simulink model "model_nonlinear_bike_closed_loop"  (R2018b)
settings: Solver=VariableStepAuto  StartTime=0.0  StopTime=60  RelTol=1e-3
values from neighbouring files (symbols this model uses):
  bike =     [bike.mat]    (also in modelconfig.mat)
  controller =     [modelconfig.mat]
  model_settings =     [modelconfig.mat]
  parameters =     [modelconfig.mat]
  state_space =     [modelconfig.mat]
undefined symbols (not defined in the file or in its folder): Continuous, Noise, observer, Time
libraries: dspindex x1, sharedTrackingLibrary x1, ctrlSharedLib x1
settings Model: Creator=micha  LastModifiedBy=mekat

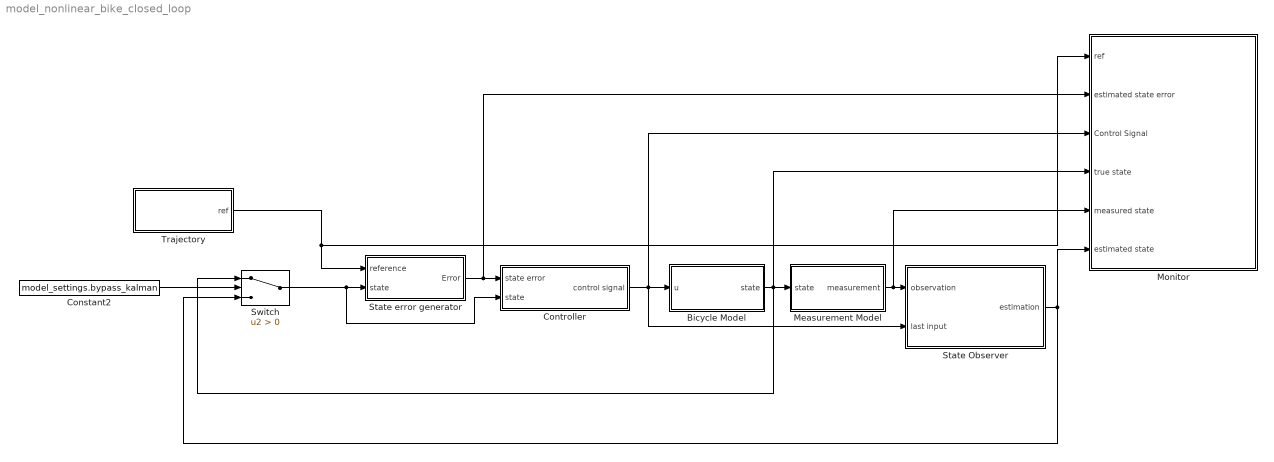
== system model_nonlinear_bike_closed_loop ==
  Bicycle Model : Subsystem
  Constant2 : Constant  Value=model_settings.bypass_kalman
  Controller : Subsystem
  Measurement Model : Subsystem
  Monitor : Subsystem
  State Observer : Subsystem
  State error generator : Subsystem
  Switch : Switch  Criteria=u2 > Threshold
  Trajectory : Subsystem
  wires:
  Bicycle Model/1(state) -> Switch/1, Monitor/4(true state), Measurement Model/1(state)
  Measurement Model/1(measurement) -> Monitor/5(measured state), State Observer/1(observation)
  Controller/1(control signal) -> Bicycle Model/1(u), State Observer/2(last input), Monitor/3(Control Signal)
  State Observer/1(estimation) -> Monitor/6(estimated state), Switch/3
  State error generator/1(Error) -> Controller/1(state error), Monitor/2(estimated state error)
  Trajectory/1(ref) -> State error generator/1(reference), Monitor/1(ref)
  Constant2/1 -> Switch/2
  Switch/1 -> Controller/2(state), State error generator/2(state)

== system model_nonlinear_bike_closed_loop/Bicycle Model ==
  u : Inport
  Constant : Constant  Commented=on  Value=model_settings.limit_model_states
  Nonlinear Model : Subsystem  Commented=on
  Nonlinear Model with Limits : Subsystem
  Switch : Switch  Commented=on  Criteria=u2 > Threshold
  state : Outport
  wires:
  Nonlinear Model with Limits/1(state) -> state/1
  Constant/1 -> Switch/2
  Switch/1 -> ?
  u/1 -> Nonlinear Model with Limits/1(u)

== system model_nonlinear_bike_closed_loop/Controller ==
  state error : Inport
  state : Inport  Port=2
  Constant : Constant  Value=model_settings.use_static_controller
  Dynamic controller : Subsystem
  Static controller : Subsystem
  Switch : Switch  Criteria=u2 > Threshold
  control signal : Outport
  wires:
  state error/1 -> Static controller/1(In1), Dynamic controller/1(stateError)
  Static controller/1(Out1) -> Switch/1
  Dynamic controller/1(control signal) -> Switch/3
  Switch/1 -> control signal/1
  Constant/1 -> Switch/2
  state/1 -> Dynamic controller/2(state)

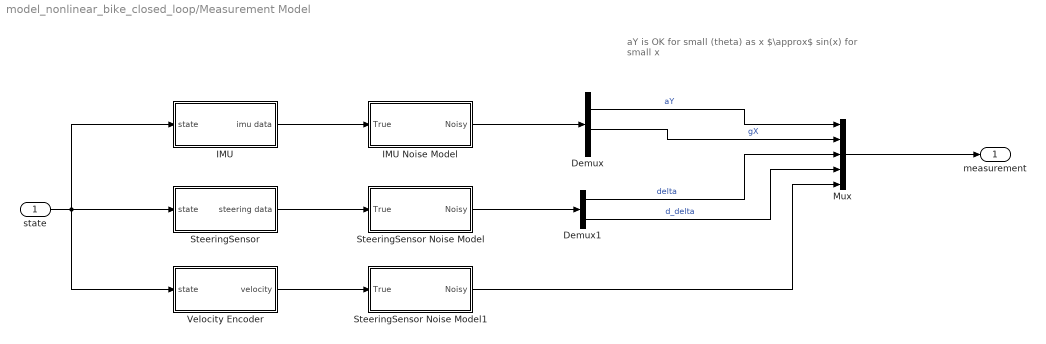
== system model_nonlinear_bike_closed_loop/Measurement Model ==
  note: aY is OK for small (theta) as x $\approx$ sin(x) for small x
  state : Inport
  Demux : Demux  Outputs=6
  Demux1 : Demux  Outputs=2
  IMU : Subsystem
  IMU Noise Model : Subsystem
  Mux : Mux  Inputs=5
  SteeringSensor : Subsystem
  SteeringSensor Noise Model : Subsystem
  SteeringSensor Noise Model1 : Subsystem
  Velocity Encoder : Subsystem
  measurement : Outport
  wires:
  state/1 -> IMU/1(state), Velocity Encoder/1(state), SteeringSensor/1(state)
  IMU/1(imu data) -> IMU Noise Model/1(True)
  SteeringSensor/1(steering data) -> SteeringSensor Noise Model/1(True)
  Demux/4 -> Mux/2  "gX"
  Demux/2 -> Mux/1  "aY"
  Demux1/1 -> Mux/3  "delta"
  Demux1/2 -> Mux/4  "d_delta"
  Mux/1 -> measurement/1
  IMU Noise Model/1(Noisy) -> Demux/1
  SteeringSensor Noise Model/1(Noisy) -> Demux1/1
  Velocity Encoder/1(velocity) -> SteeringSensor Noise Model1/1(True)
  SteeringSensor Noise Model1/1(Noisy) -> Mux/5

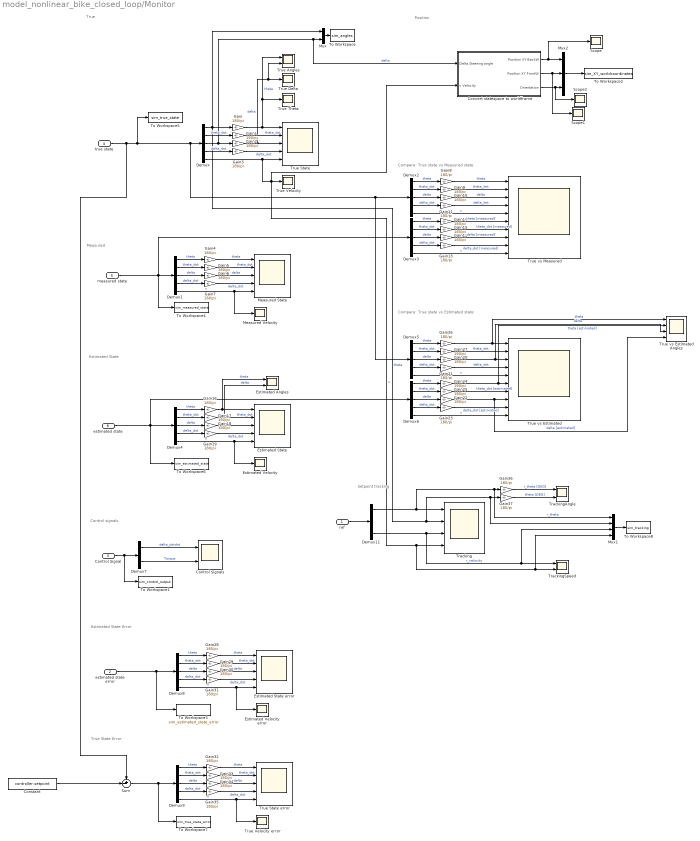
== system model_nonlinear_bike_closed_loop/Monitor ==
  note: Setpoint tracking
  note: Position
  note: Control signals
  note: Estimated State
  note: Compare: True state vs Measured state
  note: True
  note: Measured
  note: Compare: True state vs Estimated state
  note: Estimated State Error
  note: True State Error
  ref : Inport
  estimated state error : Inport  Port=2
  Control Signal : Inport  Port=3
  true state : Inport  Port=4
  measured state : Inport  Port=5
  estimated state : Inport  Port=6
  Constant : Constant  Value=controller.setpoint
  Control Signals : Scope  NumInputPorts=2
  Convert statespace to worldframe : Subsystem
  Demux{,1..6,8..9,11} (10 alike) : Demux  Outputs=5
  Demux7 : Demux  Outputs=2
  Estimated Angles : Scope  NumInputPorts=2
  Estimated State : Scope  NumInputPorts=5
  Estimated State error : Scope  NumInputPorts=5
  Estimated Velocity : Scope
  Estimated Velocity error : Scope
  Gain{,1..37} (38 alike) : Gain  Gain=180/pi
  Measured State : Scope  NumInputPorts=5
  Measured Velocity : Scope
  Mux : Mux  Inputs=2
  Mux1 : Mux
  Mux2 : Mux  Inputs=3
  Scope : Scope
  Scope1 : Scope
  Scope2 : Scope
  Sum : Sum  Inputs=+-|
  To Workspace : ToWorkspace  VariableName=sim_angles  SaveFormat=Structure With Time  SampleTime=-1
  To Workspace1 : ToWorkspace  VariableName=sim_control_output  SaveFormat=Structure With Time  SampleTime=-1
  To Workspace2 : ToWorkspace  VariableName=sim_XY_worldcoordinates  SaveFormat=Structure With Time  SampleTime=-1
  To Workspace3 : ToWorkspace  VariableName=sim_estimated_state_error  SaveFormat=Structure With Time  SampleTime=-1
  To Workspace4 : ToWorkspace  VariableName=sim_measured_state  SaveFormat=Structure With Time  SampleTime=-1
  To Workspace5 : ToWorkspace  VariableName=sim_true_state  SaveFormat=Structure With Time  SampleTime=-1
  To Workspace6 : ToWorkspace  VariableName=sim_estimated_state  SaveFormat=Structure With Time  SampleTime=-1
  To Workspace7 : ToWorkspace  VariableName=sim_true_state_error  SaveFormat=Structure With Time  SampleTime=-1
  To Workspace8 : ToWorkspace  VariableName=sim_tracking  SaveFormat=Structure With Time  SampleTime=-1
  Tracking : Scope  NumInputPorts=4
  TrackingAngle : Scope  NumInputPorts=2
  TrackingSpeed : Scope  NumInputPorts=2
  True Angles : Scope  NumInputPorts=2
  True Delta : Scope
  True State : Scope  NumInputPorts=5
  True State error : Scope  NumInputPorts=5
  True Theta : Scope
  True Velocity : Scope
  True Velocity error : Scope
  True vs Estimated : Scope  NumInputPorts=10
  True vs Estimated Angles : Scope  NumInputPorts=4
  True vs Measured : Scope  NumInputPorts=10
  wires:
  Demux/3 -> Convert statespace to worldframe/1(Delta Steering angle), Mux/2, Gain2/1  "delta"
  Gain3/1 -> True State/4  "delta_dot"
  Demux/4 -> Gain3/1  "delta_dot"
  Demux/2 -> Gain1/1  "theta_dot"
  Demux/5 -> Mux1/4, TrackingSpeed/2, Tracking/4, Convert statespace to worldframe/2(v Velocity), True Velocity/1, True State/5  "v"
  Gain/1 -> True Angles/1, True Theta/1, True State/1  "theta"
  Gain1/1 -> True State/2  "theta_dot"
  Demux/1 -> Mux1/2, Gain37/1, Tracking/2, Mux/1, Gain/1  "theta"
  Gain2/1 -> True Angles/2, True Delta/1, True State/3  "delta"
  Demux1/4 -> Gain7/1  "delta_dot"
  Demux1/3 -> Gain6/1  "delta"
  Gain7/1 -> Measured State/4  "delta_dot"
  Gain6/1 -> Measured State/3  "delta"
  Gain4/1 -> Measured State/1  "theta"
  Demux1/5 -> Measured Velocity/1, Measured State/5  "v"
  Demux1/1 -> Gain4/1  "theta"
  Demux1/2 -> Gain5/1  "theta_dot"
  Gain5/1 -> Measured State/2  "theta_dot"
  Demux2/4 -> Gain11/1  "delta_dot"
  Demux2/3 -> Gain10/1  "delta"
  Gain11/1 -> True vs Measured/4  "delta_dot"
  true state/1 -> Sum/1, To Workspace5/1, Demux5/1, Demux2/1, Demux/1
  Gain10/1 -> True vs Measured/3  "delta"
  Gain8/1 -> True vs Measured/1  "theta"
  Demux2/5 -> True vs Measured/5  "v"
  Demux2/1 -> Gain8/1  "theta"
  Demux2/2 -> Gain9/1  "theta_dot"
  Gain9/1 -> True vs Measured/2  "theta_dot"
  measured state/1 -> To Workspace4/1, Demux3/1, Demux1/1
  Gain14/1 -> True vs Measured/6  "theta [measured]"
  Gain13/1 -> True vs Measured/9  "delta_dot [measured]"
  Demux3/3 -> Gain12/1  "delta"
  Gain12/1 -> True vs Measured/8  "delta [measured]"
  Gain15/1 -> True vs Measured/7  "theta_dot [measured]"
  Demux3/4 -> Gain13/1  "delta_dot"
  Demux3/2 -> Gain15/1  "theta_dot"
  Demux3/1 -> Gain14/1  "theta"
  Demux3/5 -> True vs Measured/10  "v"
  Gain16/1 -> Estimated Angles/1, Estimated State/1  "theta"
  Gain19/1 -> Estimated State/4  "delta_dot"
  Demux4/4 -> Gain19/1  "delta_dot"
  Demux4/1 -> Gain16/1  "theta"
  Gain17/1 -> Estimated State/2  "theta_dot"
  Demux4/3 -> Gain18/1  "delta"
  Demux4/5 -> Estimated Velocity/1, Estimated State/5  "v"
  Gain18/1 -> Estimated Angles/2, Estimated State/3  "delta"
  Demux4/2 -> Gain17/1  "theta_dot"
  Demux6/1 -> Gain24/1  "theta"
  Demux6/3 -> Gain22/1  "delta"
  Gain24/1 -> True vs Estimated Angles/2, True vs Estimated/6  "theta [estimated]"
  Gain20/1 -> True vs Estimated Angles/3, True vs Estimated/3  "delta"
  Gain21/1 -> True vs Estimated/4  "delta_dot"
  Gain26/1 -> True vs Estimated/1, True vs Estimated Angles/1  "theta"
  Demux5/5 -> True vs Estimated/5  "v"
  Gain27/1 -> True vs Estimated/2  "theta_dot"
  Demux5/3 -> Gain20/1  "delta"
  Demux5/4 -> Gain21/1  "delta_dot"
  Demux5/2 -> Gain27/1  "theta_dot"
  Demux6/5 -> True vs Estimated/10  "v"
  Demux5/1 -> Gain26/1  "theta"
  Gain22/1 -> True vs Estimated Angles/4, True vs Estimated/8  "delta [estimated]"
  Demux6/4 -> Gain23/1  "delta_dot"
  Gain25/1 -> True vs Estimated/7  "theta_dot [estimated]"
  Demux6/2 -> Gain25/1  "theta_dot"
  Gain23/1 -> True vs Estimated/9  "delta_dot [estimated]"
  estimated state/1 -> Demux6/1, To Workspace6/1, Demux4/1
  Control Signal/1 -> To Workspace1/1, Demux7/1
  Demux7/1 -> Control Signals/1  "delta_dotdot"
  Demux7/2 -> Control Signals/2  "Torque"
  Gain30/1 -> Estimated State error/3  "delta"
  Demux8/2 -> Gain29/1  "theta_dot"
  Demux8/3 -> Gain30/1  "delta"
  Gain31/1 -> Estimated State error/4  "delta_dot"
  Demux8/5 -> Estimated Velocity error/1, Estimated State error/5  "v"
  Demux8/1 -> Gain28/1  "theta"
  Demux8/4 -> Gain31/1  "delta_dot"
  Gain28/1 -> Estimated State error/1  "theta"
  estimated state error/1 -> To Workspace3/1, Demux8/1
  Gain29/1 -> Estimated State error/2  "theta_dot"
  Demux9/1 -> Gain32/1  "theta"
  Demux9/4 -> Gain35/1  "delta_dot"
  Gain32/1 -> True State error/1  "theta"
  Demux9/5 -> True Velocity error/1, True State error/5  "v"
  Sum/1 -> To Workspace7/1, Demux9/1
  Demux9/2 -> Gain33/1  "theta_dot"
  Gain33/1 -> True State error/2  "theta_dot"
  Gain35/1 -> True State error/4  "delta_dot"
  Demux9/3 -> Gain34/1  "delta"
  Gain34/1 -> True State error/3  "delta"
  Constant/1 -> Sum/2
  Mux/1 -> To Workspace/1
  ref/1 -> Demux11/1
  Demux11/1 -> Mux1/1, Gain36/1, Tracking/1  "r_theta"
  Demux11/5 -> Mux1/3, TrackingSpeed/1, Tracking/3  "r_velocity"
  Gain36/1 -> TrackingAngle/1  "r_theta [DEG]"
  Gain37/1 -> TrackingAngle/2  "theta [DEG]"
  Mux1/1 -> To Workspace8/1
  Convert statespace to worldframe/3(Orientation) -> Scope2/1, Mux2/3
  Convert statespace to worldframe/2(Position XY FrontW) -> Scope1/1, Mux2/2
  Convert statespace to worldframe/1(Position XY BackW) -> Scope/1, Mux2/1
  Mux2/1 -> To Workspace2/1

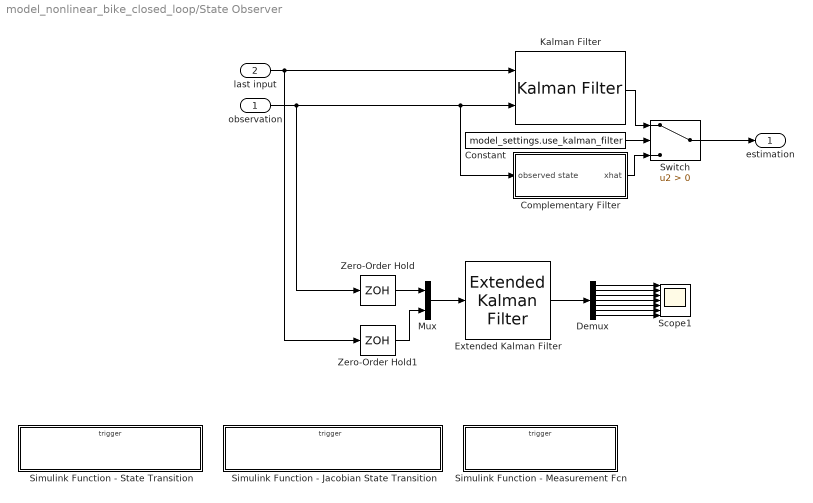
== system model_nonlinear_bike_closed_loop/State Observer ==
  observation : Inport
  last input : Inport  Port=2
  Complementary Filter : Subsystem
  Constant : Constant  Value=model_settings.use_kalman_filter
  Demux : Demux  Outputs=7
  Extended Kalman Filter : sharedTrackingLibrary/Extended Kalman Filter  StateTransitionFcn=stateTransitionFcn  HasStateTransitionJacobianFcn=on  StateTransitionJacobianFcn=JacobianStateTransitionFcn  HasAdditiveProcessNoise=Additive  ProcessNoise=EKF.Noise.stateEstimate  HasTimeVaryingProcessNoise=off  HasStateTransitionFcnExtraArgument=0  InitialState=EKF.InitialPoint  InitialStateCovariance=EKF.Noise.InitialPoint  MeasurementFcn1=measurementFcn  HasMeasurementJacobianFcn1=off  HasMeasurementEnablePort1=off  HasAdditiveMeasurementNoise1=Additive  MeasurementNoise1=EKF.Noise.measurement  HasTimeVaryingMeasurementNoise1=off  HasMeasurementFcnExtraArgument1=0  MeasurementFcn2=myMeasurementFcn  HasMeasurementJacobianFcn2=off  HasMeasurementEnablePort2=off  HasAdditiveMeasurementNoise2=Additive  MeasurementNoise2=1  HasTimeVaryingMeasurementNoise2=off  HasMeasurementFcnExtraArgument2=0  MeasurementFcn3=myMeasurementFcn  HasMeasurementJacobianFcn3=off  HasMeasurementEnablePort3=off  HasAdditiveMeasurementNoise3=Additive  MeasurementNoise3=1  HasTimeVaryingMeasurementNoise3=off  HasMeasurementFcnExtraArgument3=0  MeasurementFcn4=myMeasurementFcn  HasMeasurementJacobianFcn4=off  HasMeasurementEnablePort4=off  HasAdditiveMeasurementNoise4=Additive  MeasurementNoise4=1  HasTimeVaryingMeasurementNoise4=off  HasMeasurementFcnExtraArgument4=0  MeasurementFcn5=myMeasurementFcn  HasMeasurementJacobianFcn5=off  HasMeasurementEnablePort5=off  HasAdditiveMeasurementNoise5=Additive  MeasurementNoise5=1  HasTimeVaryingMeasurementNoise5=off  HasMeasurementFcnExtraArgument5=0  EnableMultirate=off  StateTransitionFcnSampleTime=1  MeasurementFcn1SampleTime=1  MeasurementFcn2SampleTime=1  MeasurementFcn3SampleTime=1  MeasurementFcn4SampleTime=1  MeasurementFcn5SampleTime=1  UseCurrentEstimator=on  OutputStateCovariance=off  DataType=double  SampleTime=parameters.Ts  NumberOfMeasurements=1
      settings: SourceProductName=Control System Toolbox  SourceProductBaseCode=CT
  Kalman Filter : ctrlSharedLib/Kalman Filter  TimeDomain=Continuous-Time  UseCurrentEstimator=on  ModelSource=Individual A, B, C, D matrices  ModelSourceVariable=ss(0.95,1,1,0,1)  A=state_space.A  B=state_space.B  C=state_space.C  D=state_space.D  NumberOfStates=1  NumberOfInputs=1  NumberOfOutputs=1  InitialEstimateSource=Dialog  X0=state_space.x0  P0=10  UseK=off  UseGH=off  NumberOfProcessNoiseInputs=1  G=1  TimeInvariantG=on  H=0  TimeInvariantH=on  Q=observer.Q  TimeInvariantQ=on  R=observer.R  TimeInvariantR=on  N=0  TimeInvariantN=on  AddInputPort=on  AddEnablePort=off  OutputEstimatedY=off  OutputP=off  Ts=-1
      settings: SourceProductBaseCode=CT
  Mux : Mux  Inputs=2
  Scope1 : Scope  NumInputPorts=7
  "Simulink Function - Jacobian State Transition " : Subsystem  TreatAsAtomicUnit=on
  Simulink Function - Measurement Fcn : Subsystem  TreatAsAtomicUnit=on
  Simulink Function - State Transition : Subsystem  TreatAsAtomicUnit=on
  Switch : Switch  Criteria=u2 > Threshold
  Zero-Order Hold : ZeroOrderHold  SampleTime=parameters.Ts
  Zero-Order Hold1 : ZeroOrderHold  SampleTime=parameters.Ts
  estimation : Outport
  wires:
  observation/1 -> Zero-Order Hold/1, Kalman Filter/2, Complementary Filter/1(observed state)
  last input/1 -> Zero-Order Hold1/1, Kalman Filter/1
  Switch/1 -> estimation/1
  Kalman Filter/1 -> Switch/1
  Complementary Filter/1(xhat) -> Switch/3
  Constant/1 -> Switch/2
  Demux/2 -> Scope1/2
  Demux/4 -> Scope1/4
  Demux/5 -> Scope1/5
  Demux/3 -> Scope1/3
  Demux/1 -> Scope1/1
  Extended Kalman Filter/1 -> Demux/1
  Zero-Order Hold/1 -> Mux/1
  Zero-Order Hold1/1 -> Mux/2
  Mux/1 -> Extended Kalman Filter/1
  Demux/6 -> Scope1/6
  Demux/7 -> Scope1/7

== system model_nonlinear_bike_closed_loop/State error generator ==
  reference : Inport
  state : Inport  Port=2
  Sum : Sum  Inputs=|-+
  Error : Outport
  wires:
  reference/1 -> Sum/1
  Sum/1 -> Error/1
  state/1 -> Sum/2

== system model_nonlinear_bike_closed_loop/Trajectory ==
  Clock : Clock
  Constant : Constant  Value=model_settings.SpeedProfile
  Constant1 : Constant  Value=0
  Constant2 : Constant  Value=state_space.x0(5)
  MATLAB Function : MATLAB Function  TreatAsAtomicUnit=on
  Mux : Mux  Inputs=5
  ref : Outport
  wires:
  Mux/1 -> ref/1
  Constant1/1 -> Mux/4, Mux/3, Mux/2, Mux/1
  Clock/1 -> MATLAB Function/1(t)
  MATLAB Function/1(v) -> Mux/5
  Constant/1 -> MATLAB Function/2(t_case)
  Constant2/1 -> MATLAB Function/3(v0)

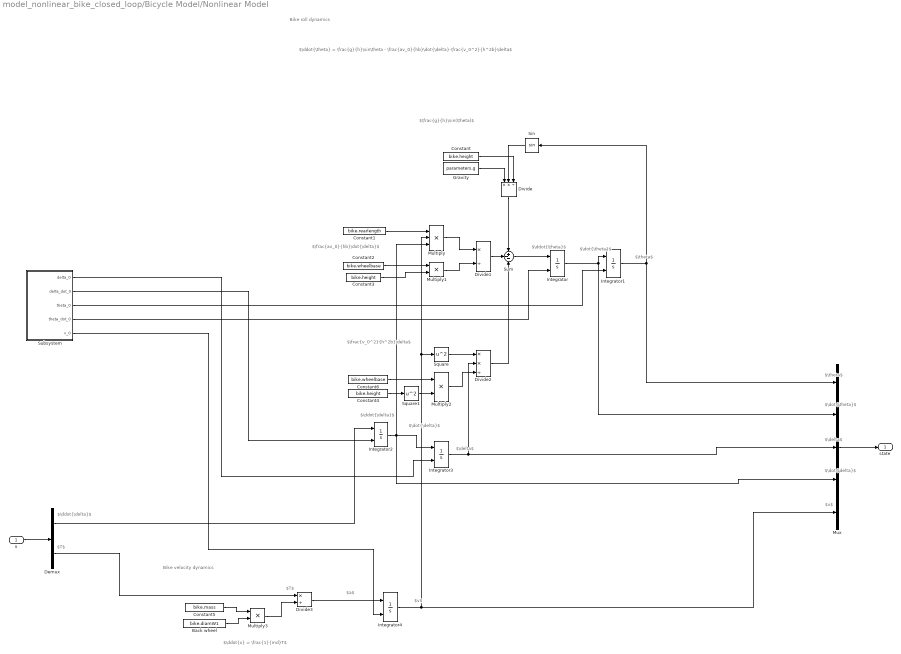
== system model_nonlinear_bike_closed_loop/Bicycle Model/Nonlinear Model ==
  note: Bike velocity dynamics
  note: $\ddot{\theta} = \frac{g}{h}\sin\theta - \frac{av_0}{hb}\dot{\delta}-\frac{v_0^2}{h^2b}\delta$
  note: Bike roll dynamics
  note: $\ddot{x} = \frac{1}{md}T$
  note: $T$
  note: $v$
  note: $a$
  note: $\frac{v_0^2}{h^2b}\delta$
  note: $\frac{g}{h}\sin(\theta)$
  note: $\frac{av_0}{hb}\dot{\delta}$
  note: $\delta$
  note: $\dot{\delta}$
  note: $\ddot{\delta}$
  note: $\theta$
  note: $\dot{\theta}$
  note: $\ddot{\theta}$
  note: $\theta$
  note: $\dot{\theta}$
  note: $\delta$
  note: $\dot{\delta}$
  note: $v$
  note: $\ddot{\delta}$
  note: $T$
  u : Inport
  Back wheel : Constant  Value=bike.diamW1
  Constant : Constant  Value=bike.height
  Constant1 : Constant  Value=bike.rearlength
  Constant2 : Constant  Value=bike.wheelbase
  Constant3 : Constant  Value=bike.height
  Constant4 : Constant  Value=bike.height
  Constant5 : Constant  Value=bike.mass
  Constant6 : Constant  Value=bike.wheelbase
  Demux : Demux  Outputs=2
  Divide : Product  Inputs=**/
  Divide1 : Product  Inputs=*/
  Divide2 : Product  Inputs=**/
  Divide3 : Product  Inputs=*/
  Gravity : Constant  Value=parameters.g
  Integrator{,1..4} (5 alike) : Integrator  InitialConditionSource=external
  Multiply : Product  Inputs=3
  Multiply1 : Product
  Multiply2 : Product
  Multiply3 : Product
  Mux : Mux  Inputs=5
  Sin : Trigonometry
  Square : Math  Operator=square  SaturateOnIntegerOverflow=on
  Square1 : Math  Operator=square  SaturateOnIntegerOverflow=on
  Subsystem : Subsystem
  Sum : Sum  Inputs=+--
  state : Outport
  wires:
  Integrator/1 -> Integrator1/1, Mux/2
  Integrator1/1 -> Mux/1, Sin/1
  Sum/1 -> Integrator/1
  Divide/1 -> Sum/1
  Gravity/1 -> Divide/1
  Sin/1 -> Divide/2
  Constant/1 -> Divide/3
  Demux/1 -> Integrator2/1
  Integrator2/1 -> Integrator3/1, Mux/4, Multiply/3
  Integrator3/1 -> Mux/3, Divide2/2
  Divide1/1 -> Sum/2
  Multiply/1 -> Divide1/1
  Multiply1/1 -> Divide1/2
  Constant1/1 -> Multiply/1
  Constant2/1 -> Multiply1/1
  Constant3/1 -> Multiply1/2
  Divide2/1 -> Sum/3
  Multiply2/1 -> Divide2/3
  Constant4/1 -> Square1/1
  Constant6/1 -> Multiply2/1
  Mux/1 -> state/1
  u/1 -> Demux/1
  Integrator4/1 -> Multiply/2, Square/1, Mux/5
  Square/1 -> Divide2/1
  Square1/1 -> Multiply2/2
  Demux/2 -> Divide3/1
  Multiply3/1 -> Divide3/2
  Constant5/1 -> Multiply3/1
  Back wheel/1 -> Multiply3/2
  Divide3/1 -> Integrator4/1
  Subsystem/3(theta_0) -> Integrator1/2
  Subsystem/4(theta_dot_0) -> Integrator/2
  Subsystem/2(delta_dot_0) -> Integrator2/2
  Subsystem/1(delta_0) -> Integrator3/2
  Subsystem/5(v_0) -> Integrator4/2

== system model_nonlinear_bike_closed_loop/Bicycle Model/Nonlinear Model with Limits ==
  note: $\theta$
  note: $\dot{\theta}$
  note: $\delta$
  note: $\dot{\delta}$
  note: $v$
  note: $\ddot{\delta}$
  note: $T$
  u : Inport
  Demux : Demux  Outputs=2
  Mux : Mux  Inputs=5
  Roll Dynamics : Subsystem
  Velocity Dynamics : Subsystem
  state : Outport
  wires:
  Mux/1 -> state/1
  u/1 -> Demux/1
  Demux/1 -> Roll Dynamics/2(delta_dot_dot)
  Roll Dynamics/1(theta) -> Mux/1
  Roll Dynamics/2(theta_dot) -> Mux/2
  Roll Dynamics/3(delta) -> Mux/3
  Roll Dynamics/4(delta_dot) -> Mux/4
  Velocity Dynamics/1(v) -> Roll Dynamics/1(v), Mux/5
  Demux/2 -> Velocity Dynamics/1(T)

== system model_nonlinear_bike_closed_loop/Controller/Dynamic controller ==
  note: These two blocks implement the same controller.
      | The simulink implementation was made in the hopes that
      | it would be faster.
  stateError : Inport
  state : Inport  Port=2
  Constant : Constant  Value=controller.vmin
  Constant1 : Constant  Value=controller.vmax
  Constant2 : Constant  Value=model_settings.simulink_implementation
  MATLAB Function : MATLAB Function  TreatAsAtomicUnit=on
  Simulink implementation : Subsystem
  Switch : Switch  Criteria=u2 > Threshold
  control signal : Outport
  wires:
  stateError/1 -> Simulink implementation/2(state_error), MATLAB Function/3(state)
  MATLAB Function/1(feedback) -> Switch/3
  Constant/1 -> Simulink implementation/3(vmin), MATLAB Function/1(vmin)
  Constant1/1 -> Simulink implementation/4(vmax), MATLAB Function/2(vmax)
  Constant2/1 -> Switch/2
  Simulink implementation/1(feedback) -> Switch/1
  Switch/1 -> control signal/1
  state/1 -> Simulink implementation/1(state)

== system model_nonlinear_bike_closed_loop/Controller/Static controller ==
  In1 : Inport
  Gain : Gain  Gain=-controller.K  Multiplication=Matrix(K*u)
  Out1 : Outport
  wires:
  Gain/1 -> Out1/1
  In1/1 -> Gain/1

== system model_nonlinear_bike_closed_loop/Measurement Model/IMU ==
  state : Inport
  Accelerometer : Subsystem
  Gyroscope : Subsystem
  Mux : Mux  Inputs=2
  imu data : Outport
  wires:
  state/1 -> Gyroscope/1(state), Accelerometer/1(state)
  Mux/1 -> imu data/1
  Accelerometer/1(acceleration) -> Mux/1  "acc"
  Gyroscope/1(gyro) -> Mux/2  "gyro"

== system model_nonlinear_bike_closed_loop/Measurement Model/IMU Noise Model ==
  note: Generate additive noise
  True : Inport
  Constant1 : Constant  Value=zeros(6,1)
  Constant2 : Constant  Value=model_settings.enable_imu_noise
  Noise Covariance : Gain  Gain=Noise.IMU  Multiplication=Matrix(K*u)
  Random Gaussian : RandomNumber  Seed=round(100000*rand(6,1))  SampleTime=0.02
  Sum : Sum  Inputs=|++
  Switch : Switch  Criteria=u2 > Threshold
  Noisy : Outport
  wires:
  Random Gaussian/1 -> Switch/1
  Switch/1 -> Noise Covariance/1
  Constant2/1 -> Switch/2
  Constant1/1 -> Switch/3
  Noise Covariance/1 -> Sum/2
  True/1 -> Sum/1
  Sum/1 -> Noisy/1

== system model_nonlinear_bike_closed_loop/Measurement Model/SteeringSensor ==
  state : Inport
  Demux : Demux  Outputs=5
  Mux : Mux  Inputs=2
  steering data : Outport
  wires:
  state/1 -> Demux/1
  Mux/1 -> steering data/1
  Demux/3 -> Mux/1  "delta"
  Demux/4 -> Mux/2  "d_delta"

== system model_nonlinear_bike_closed_loop/Measurement Model/SteeringSensor Noise Model ==
  note: Generate additive noise
  True : Inport
  Constant1 : Constant  Value=zeros(2,1)
  Constant2 : Constant  Value=model_settings.enable_encoder_noise
  Noise Covariance : Gain  Gain=Noise.steering_encoder_noise  Multiplication=Matrix(K*u)
  Random Gaussian : RandomNumber  Seed=round(100000*rand(2,1))  SampleTime=0.02
  Sum : Sum  Inputs=-+|
  Switch : Switch  Criteria=u2 > Threshold
  Noisy : Outport
  wires:
  True/1 -> Sum/2
  Switch/1 -> Noise Covariance/1
  Constant1/1 -> Switch/3
  Constant2/1 -> Switch/2
  Random Gaussian/1 -> Switch/1
  Sum/1 -> Noisy/1
  Noise Covariance/1 -> Sum/1

== system model_nonlinear_bike_closed_loop/Measurement Model/SteeringSensor Noise Model1 ==
  note: Generate additive noise
  True : Inport
  Constant1 : Constant  Value=zeros(1,1)
  Constant2 : Constant  Value=model_settings.enable_velocity_noise
  Noise Covariance : Gain  Gain=Noise.velocity_sensor  Multiplication=Matrix(K*u)
  Random Gaussian : RandomNumber  Seed=round(100000*rand(1,1))  SampleTime=0.02
  Sum : Sum  Inputs=-+|
  Switch : Switch  Criteria=u2 > Threshold
  Noisy : Outport
  wires:
  True/1 -> Sum/2
  Switch/1 -> Noise Covariance/1
  Constant1/1 -> Switch/3
  Constant2/1 -> Switch/2
  Random Gaussian/1 -> Switch/1
  Sum/1 -> Noisy/1
  Noise Covariance/1 -> Sum/1

== system model_nonlinear_bike_closed_loop/Measurement Model/Velocity Encoder ==
  state : Inport
  Demux : Demux  Outputs=5
  velocity : Outport
  wires:
  state/1 -> Demux/1
  Demux/5 -> velocity/1

== system model_nonlinear_bike_closed_loop/Monitor/Convert statespace to worldframe ==
  note: This is a forward kinematic system that calculates the
      | velocity in the bikes internal frame and then is
      | transformed (rotated and "translated") into the
      | world frame X and Y.
      | Here to simplify, the orientation is assumed to be
      | the integration of the steering angle.
      | Assumes that bike starts with backwheel in origo and frontwheel on x-axis
  Delta Steering angle : Inport
  v Velocity : Inport  Port=2
  Convert Statespace to World frame : MATLAB Function  TreatAsAtomicUnit=on
  MATLAB Function : MATLAB Function  TreatAsAtomicUnit=on
  Position1 : Integrator  InitialConditionSource=external  InitialCondition=[0,0]'  ContinuousStateAttributes='Position_Global'
  StartingPos Frontwheel : Constant  Value=[bike.wheelbase,0]'
  "orientation " : Integrator  ContinuousStateAttributes='Orientation'
  Position XY BackW : Outport
  Position XY FrontW : Outport  Port=2
  Orientation : Outport  Port=3
  wires:
  "orientation "/1 -> Orientation/1, MATLAB Function/1(orientation), Convert Statespace to World frame/1(orientation_n)
  Delta Steering angle/1 -> Convert Statespace to World frame/2(delta), "orientation "/1
  v Velocity/1 -> Convert Statespace to World frame/3(velocity)
  Convert Statespace to World frame/1(Vel_FW) -> Position1/1
  Position1/1 -> Position XY FrontW/1, MATLAB Function/2(Pos_frontwheel)
  StartingPos Frontwheel/1 -> Position1/2
  MATLAB Function/1(Pos_BW) -> Position XY BackW/1

== system model_nonlinear_bike_closed_loop/State Observer/Complementary Filter ==
  note: $v$
  note: $\dot{\delta}$
  note: $\delta$
  note: $\dot{\theta}$
  note: $\theta$
  observed state : Inport
  Demux : Demux  Outputs=5
  Mux : Mux  Inputs=5
  Subsystem : Subsystem
  Subsystem1 : Subsystem
  xhat : Outport
  wires:
  observed state/1 -> Demux/1
  Demux/2 -> Subsystem/2(obs.rate)
  Demux/3 -> Subsystem1/1(obs.angle)
  Demux/4 -> Subsystem1/2(obs.rate)
  Mux/1 -> xhat/1
  Demux/5 -> Mux/5
  Demux/1 -> Subsystem/1(obs.angle)
  Subsystem/1(est.angle) -> Mux/1
  Subsystem/2(est.rate) -> Mux/2
  Subsystem1/1(est.angle) -> Mux/3
  Subsystem1/2(est.rate) -> Mux/4

== system model_nonlinear_bike_closed_loop/State Observer/Simulink Function - Jacobian State Transition  ==
  JacobianStateTransitionFcn : TriggerPort  TriggerType=function-call  IsSimulinkFunction=on  FunctionName=JacobianStateTransitionFcn  VariantControl=(inherit)
  Demux : Demux  Outputs=7
  MATLAB Function : MATLAB Function  TreatAsAtomicUnit=on
  Mux : Mux  Inputs=3
  Terminator{,1..3} (4 alike) : Terminator
  x : ArgIn  DisableCoverage=on  PortDimensions=7  ArgumentName=x
  A~ : ArgOut  DisableCoverage=on  PortDimensions=[7,7]  ArgumentName=A
  wires:
  x/1 -> Demux/1
  Mux/1 -> MATLAB Function/1(xhat)
  Demux/5 -> Mux/3
  Demux/4 -> Mux/2
  Demux/3 -> Mux/1
  Demux/1 -> Terminator/1
  Demux/2 -> Terminator1/1
  Demux/7 -> Terminator3/1
  Demux/6 -> Terminator2/1
  MATLAB Function/1(A) -> A~/1

== system model_nonlinear_bike_closed_loop/State Observer/Simulink Function - Measurement Fcn ==
  measurementFcn : TriggerPort  TriggerType=function-call  IsSimulinkFunction=on  FunctionName=measurementFcn  VariantControl=(inherit)
  x : ArgIn  DisableCoverage=on  PortDimensions=7  ArgumentName=x
  y : ArgOut  DisableCoverage=on  PortDimensions=7  ArgumentName=y
  wires:
  x/1 -> y/1

== system model_nonlinear_bike_closed_loop/State Observer/Simulink Function - State Transition ==
  stateTransitionFcn : TriggerPort  TriggerType=function-call  IsSimulinkFunction=on  FunctionName=stateTransitionFcn  VariantControl=(inherit)  ShowOutputPort=on  OutputDataType=double
  MATLAB SFunction : MATLAB Function  TreatAsAtomicUnit=on
  x : ArgIn  DisableCoverage=on  PortDimensions=7  ArgumentName=x
  xNext : ArgOut  DisableCoverage=on  PortDimensions=7  ArgumentName=xNext
  wires:
  MATLAB SFunction/1(next_xhat) -> xNext/1
  x/1 -> MATLAB SFunction/1(xhat)

== system model_nonlinear_bike_closed_loop/Bicycle Model/Nonlinear Model/Subsystem ==
  Constant : Constant  Value=state_space.x0(1)
  Constant1 : Constant  Value=state_space.x0(2)
  Constant2 : Constant  Value=state_space.x0(3)
  Constant3 : Constant  Value=state_space.x0(4)
  Constant4 : Constant  Value=state_space.x0(5)
  delta_0 : Outport
  delta_dot_0 : Outport  Port=2
  theta_0 : Outport  Port=3
  theta_dot_0 : Outport  Port=4
  v_0 : Outport  Port=5
  wires:
  Constant/1 -> delta_0/1
  Constant1/1 -> delta_dot_0/1
  Constant2/1 -> theta_0/1
  Constant3/1 -> theta_dot_0/1
  Constant4/1 -> v_0/1

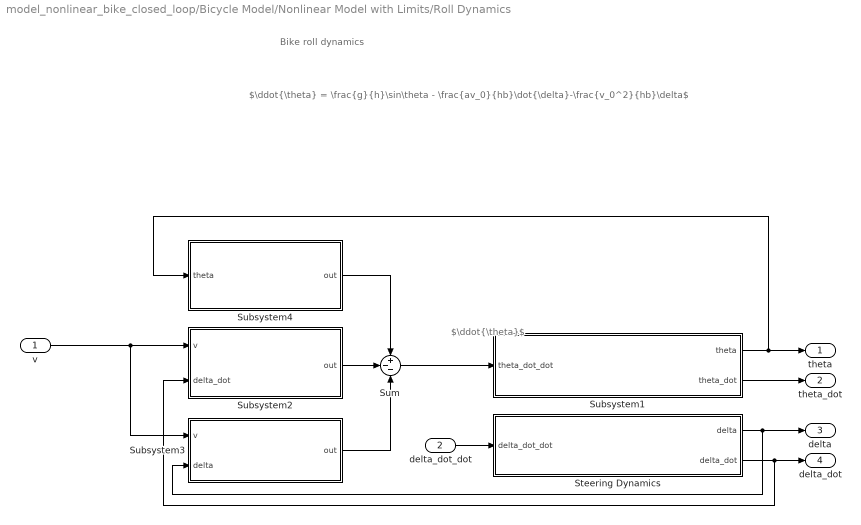
== system model_nonlinear_bike_closed_loop/Bicycle Model/Nonlinear Model with Limits/Roll Dynamics ==
  note: $\ddot{\theta}$
  note: $\ddot{\theta} = \frac{g}{h}\sin\theta - \frac{av_0}{hb}\dot{\delta}-\frac{v_0^2}{hb}\delta$
  note: Bike roll dynamics
  v : Inport
  delta_dot_dot : Inport  Port=2
  Steering Dynamics : Subsystem
  Subsystem1 : Subsystem
  Subsystem2 : Subsystem
  Subsystem3 : Subsystem
  Subsystem4 : Subsystem
  Sum : Sum  Inputs=+--
  theta : Outport
  theta_dot : Outport  Port=2
  delta : Outport  Port=3
  delta_dot : Outport  Port=4
  wires:
  Subsystem3/1(out) -> Sum/3
  v/1 -> Subsystem3/1(v), Subsystem2/1(v)
  Subsystem4/1(out) -> Sum/1
  Steering Dynamics/1(delta) -> Subsystem3/2(delta), delta/1
  Sum/1 -> Subsystem1/1(theta_dot_dot)
  Steering Dynamics/2(delta_dot) -> Subsystem2/2(delta_dot), delta_dot/1
  Subsystem1/1(theta) -> theta/1, Subsystem4/1(theta)
  Subsystem2/1(out) -> Sum/2
  Subsystem1/2(theta_dot) -> theta_dot/1
  delta_dot_dot/1 -> Steering Dynamics/1(delta_dot_dot)

== system model_nonlinear_bike_closed_loop/Bicycle Model/Nonlinear Model with Limits/Velocity Dynamics ==
  note: Bike velocity dynamics
  note: $\ddot{x} = \frac{1}{md}T - \mu_f v - F_c$
  note: $v$
  note: $a$
  T : Inport
  Subsystem : Subsystem
  Subsystem5 : Subsystem
  Subsystem6 : Subsystem
  Subsystem7 : Subsystem
  Sum1 : Sum  Inputs=+--
  v : Outport
  wires:
  Sum1/1 -> Subsystem7/1(a)
  Subsystem6/1(out) -> Sum1/2
  Subsystem/1(out) -> Sum1/1
  Subsystem5/1(out) -> Sum1/3
  T/1 -> Subsystem/1(T)
  Subsystem7/1(v) -> Subsystem6/1(v), Subsystem5/1(v), v/1

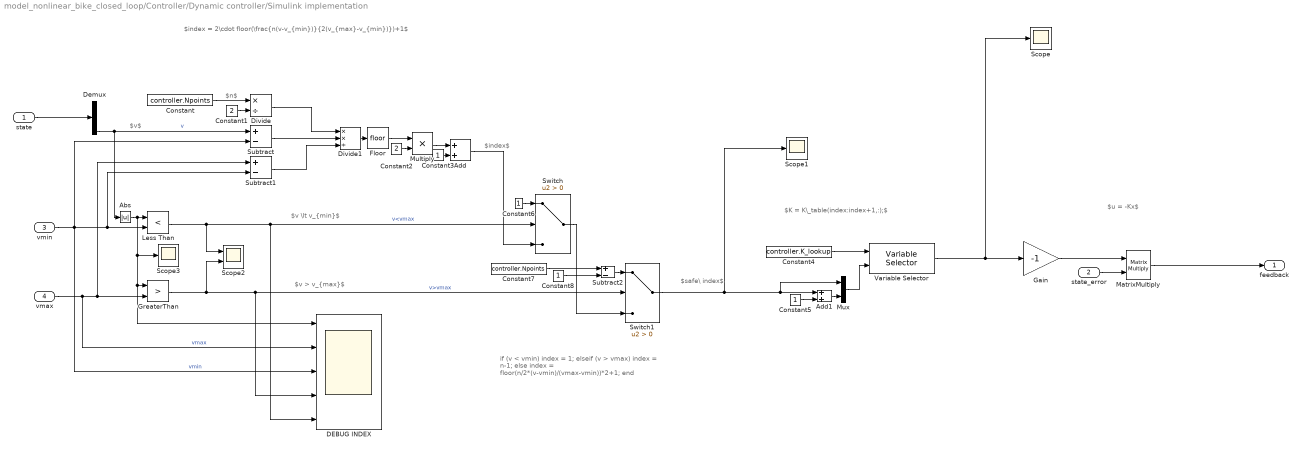
== system model_nonlinear_bike_closed_loop/Controller/Dynamic controller/Simulink implementation ==
  note: $v \lt v_{min}$
  note: if (v < vmin)
      | 	index = 1;
      | elseif (v > vmax)
      | 	index = n-1;
      | else
      | 	index = floor(n/2*(v-vmin)/(vmax-vmin))*2+1;
      | end
  note: $u = -Kx$
  note: $K = K\_table(index:index+1,:);$
  note: $safe\ index$
  note: $index$
  note: $n$
  note: $index = 2\cdot floor(\frac{n(v-v_{min})}{2(v_{max}-v_{min})})+1$
  note: $v$
  note: $v > v_{max}$
  state : Inport
  state_error : Inport  Port=2
  vmin : Inport  Port=3
  vmax : Inport  Port=4
  Abs : Abs
  Add : Sum
  Add1 : Sum
  Constant : Constant  Value=controller.Npoints
  Constant1 : Constant  Value=2
  Constant2 : Constant  Value=2
  Constant{3,5..6,8} (4 alike) : Constant
  Constant4 : Constant  Value=controller.K_lookup
  Constant7 : Constant  Value=controller.Npoints
  DEBUG INDEX : Scope  NumInputPorts=5
  Demux : Demux  Outputs=5
  Divide : Product  Inputs=*/
  Divide1 : Product  Inputs=**/
  Floor : Rounding
  Gain : Gain  Gain=-1
  GreaterThan : RelationalOperator  Operator=>  OutDataTypeStr=boolean  ZeroCross=off  RndMeth=Simplest
  Less Than : RelationalOperator  Operator=<  OutDataTypeStr=boolean  ZeroCross=off  RndMeth=Simplest
  MatrixMultiply : Product  Multiplication=Matrix(*)
  Multiply : Product
  Mux : Mux  Inputs=2
  Scope : Scope
  Scope1 : Scope
  Scope2 : Scope  NumInputPorts=2
  Scope3 : Scope
  Subtract : Sum  Inputs=+-
  Subtract1 : Sum  Inputs=+-
  Subtract2 : Sum  Inputs=+-
  Switch : Switch  Criteria=u2 > Threshold
  Switch1 : Switch  Criteria=u2 > Threshold
  Variable Selector : dspindex/Variable Selector  NumInputs=1  rowsOrCols=Rows  IdxMode=Variable  Elements=[1 3]  ZerOneIdxMode=One-based  errmode=Clip Index  FillMode=on  FillValues=0
  feedback : Outport
  wires:
  state_error/1 -> MatrixMultiply/2
  Demux/5 -> Subtract/1, Abs/1  "v"
  vmin/1 -> DEBUG INDEX/3, Less Than/2, Subtract1/2, Subtract/2  "vmin"
  vmax/1 -> DEBUG INDEX/2, GreaterThan/2, Subtract1/1  "vmax"
  Constant/1 -> Divide/1
  Constant1/1 -> Divide/2
  Subtract/1 -> Divide1/2
  Subtract1/1 -> Divide1/3
  Divide/1 -> Divide1/1
  Divide1/1 -> Floor/1
  Floor/1 -> Multiply/1
  Constant2/1 -> Multiply/2
  Multiply/1 -> Add/1
  Constant3/1 -> Add/2
  Add/1 -> Switch/3
  Less Than/1 -> Scope2/1, DEBUG INDEX/5, Switch/2  "v<vmax"
  GreaterThan/1 -> Scope2/2, DEBUG INDEX/4, Switch1/2  "v>vmax"
  Switch/1 -> Switch1/3
  Switch1/1 -> Add1/1, Mux/1, Scope1/1
  Constant4/1 -> Variable Selector/1
  Mux/1 -> Variable Selector/2
  Add1/1 -> Mux/2
  Constant5/1 -> Add1/2
  Gain/1 -> MatrixMultiply/1
  MatrixMultiply/1 -> feedback/1
  Variable Selector/1 -> Scope/1, Gain/1
  Constant6/1 -> Switch/1
  Subtract2/1 -> Switch1/1
  Constant7/1 -> Subtract2/1
  Constant8/1 -> Subtract2/2
  Abs/1 -> DEBUG INDEX/1, GreaterThan/1, Scope3/1, Less Than/1
  state/1 -> Demux/1

== system model_nonlinear_bike_closed_loop/Measurement Model/IMU/Accelerometer ==
  note: We assume level ground. This means acceleration in X caused by tilt will always be 0.
      |
      | When the bike is upright (theta = 0) we will have aY = 0. When the bike has fallen over (theta = pi/2) we should have 1G
      |     This means that aY = sin(theta)
      |
      | With the same argument we will have that
      |    aZ = cos(theta)
  state : Inport
  Demux : Demux  Outputs=5
  Mux : Mux  Inputs=3
  Sin : Trigonometry
  Sin1 : Trigonometry  Operator=cos
  ax : Constant  Value=0
  acceleration : Outport
  wires:
  Mux/1 -> acceleration/1
  state/1 -> Demux/1
  Demux/1 -> Sin1/1, Sin/1  "theta"
  ax/1 -> Mux/1  "aX"
  Sin/1 -> Mux/2  "aY"
  Sin1/1 -> Mux/3  "aZ"

== system model_nonlinear_bike_closed_loop/Measurement Model/IMU/Gyroscope ==
  state : Inport
  Constant : Constant  Value=0
  Demux : Demux  Outputs=5
  Gain : Gain
  Mux : Mux  Inputs=3
  TurnAngle to gZ : Subsystem
  gyro : Outport
  wires:
  Mux/1 -> gyro/1
  state/1 -> Demux/1
  Demux/2 -> Gain/1  "d_theta (roll rate)"
  Constant/1 -> Mux/2  "gY"
  Gain/1 -> Mux/1  "gX"
  Demux/3 -> TurnAngle to gZ/1(delta)
  TurnAngle to gZ/1(gZ) -> Mux/3

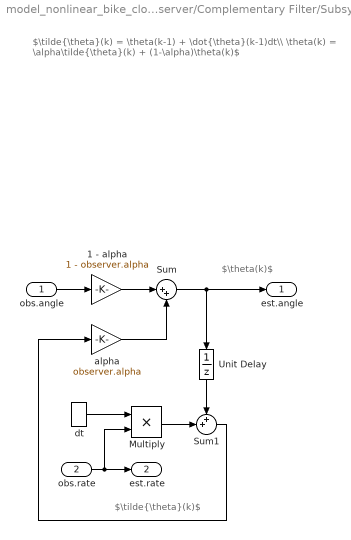
== system model_nonlinear_bike_closed_loop/State Observer/Complementary Filter/Subsystem ==
  note: $\theta(k)$
  note: $\tilde{\theta}(k)$
  note: $\tilde{\theta}(k) = \theta(k-1) + \dot{\theta}(k-1)dt\\ \theta(k) = \alpha\tilde{\theta}(k) + (1-\alpha)\theta(k)$
  obs.angle : Inport
  obs.rate : Inport  Port=2
  1 - alpha : Gain  Gain=1 - observer.alpha
  Multiply : Product
  Sum : Sum  Inputs=|++
  Sum1 : Sum  Inputs=++|
  Unit Delay : UnitDelay  SampleTime=-1
  alpha : Gain  Gain=observer.alpha
  dt : SampleTimeMath  TsampMathOp=Ts Only
  est.angle : Outport
  est.rate : Outport  Port=2
  wires:
  obs.rate/1 -> Multiply/2, est.rate/1
  Sum/1 -> Unit Delay/1, est.angle/1
  1 - alpha/1 -> Sum/1
  obs.angle/1 -> 1 - alpha/1
  alpha/1 -> Sum/2
  dt/1 -> Multiply/1
  Multiply/1 -> Sum1/2
  Unit Delay/1 -> Sum1/1
  Sum1/1 -> alpha/1

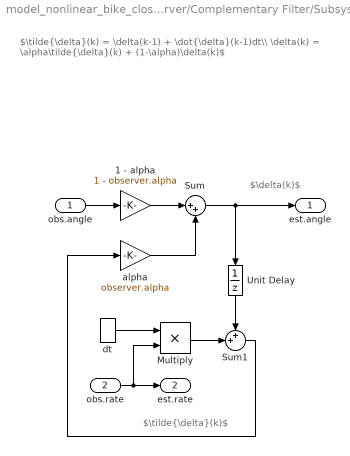
== system model_nonlinear_bike_closed_loop/State Observer/Complementary Filter/Subsystem1 ==
  note: $\delta(k)$
  note: $\tilde{\delta}(k)$
  note: $\tilde{\delta}(k) = \delta(k-1) + \dot{\delta}(k-1)dt\\ \delta(k) = \alpha\tilde{\delta}(k) + (1-\alpha)\delta(k)$
  obs.angle : Inport
  obs.rate : Inport  Port=2
  1 - alpha : Gain  Gain=1 - observer.alpha
  Multiply : Product
  Sum : Sum  Inputs=|++
  Sum1 : Sum  Inputs=++|
  Unit Delay : UnitDelay  SampleTime=-1
  alpha : Gain  Gain=observer.alpha
  dt : SampleTimeMath  TsampMathOp=Ts Only
  est.angle : Outport
  est.rate : Outport  Port=2
  wires:
  dt/1 -> Multiply/1
  Sum1/1 -> alpha/1
  1 - alpha/1 -> Sum/1
  Sum/1 -> Unit Delay/1, est.angle/1
  alpha/1 -> Sum/2
  Unit Delay/1 -> Sum1/1
  Multiply/1 -> Sum1/2
  obs.rate/1 -> Multiply/2, est.rate/1
  obs.angle/1 -> 1 - alpha/1

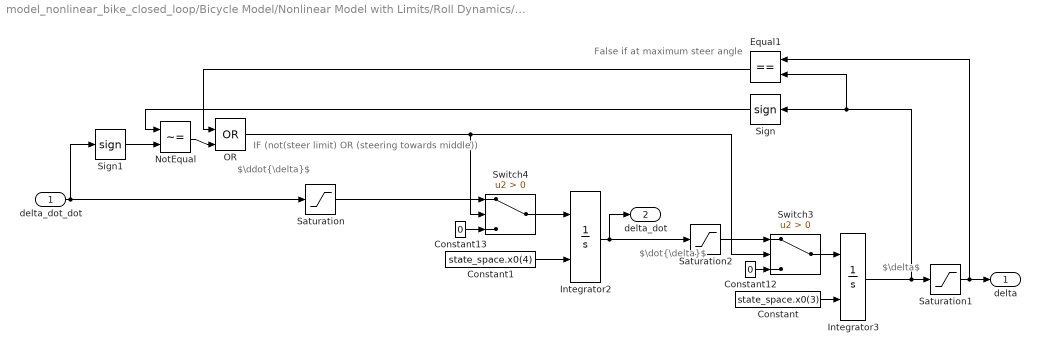
== system model_nonlinear_bike_closed_loop/Bicycle Model/Nonlinear Model with Limits/Roll Dynamics/Steering Dynamics ==
  note: IF (not(steer limit) OR (steering towards middle))
  note: False if at maximum steer angle
  note: $\delta$
  note: $\dot{\delta}$
  note: $\ddot{\delta}$
  delta_dot_dot : Inport
  Constant : Constant  Value=state_space.x0(3)
  Constant1 : Constant  Value=state_space.x0(4)
  Constant12 : Constant  Value=0
  Constant13 : Constant  Value=0
  Equal1 : RelationalOperator  Operator===  OutDataTypeStr=boolean  RndMeth=Simplest
  Integrator2 : Integrator  InitialConditionSource=external
  Integrator3 : Integrator  InitialConditionSource=external
  NotEqual : RelationalOperator  Operator=~=  OutDataTypeStr=boolean  RndMeth=Simplest
  OR : Logic  Operator=OR  IconShape=distinctive  AllPortsSameDT=off  OutDataTypeStr=boolean
  Saturation : Saturate  UpperLimit=model_settings.limit_input_max  LowerLimit=model_settings.limit_input_min  ZeroCross=off
  Saturation1 : Saturate  UpperLimit=model_settings.limit_steer_angle_max  LowerLimit=model_settings.limit_steer_angle_min  ZeroCross=off
  Saturation2 : Saturate  UpperLimit=model_settings.limit_steer_rate_max  LowerLimit=model_settings.limit_steer_rate_min  ZeroCross=off
  Sign : Signum
  Sign1 : Signum
  Switch3 : Switch  Criteria=u2 > Threshold
  Switch4 : Switch  Criteria=u2 > Threshold
  delta : Outport
  delta_dot : Outport  Port=2
  wires:
  Integrator3/1 -> Sign/1, Equal1/2, Saturation1/1
  Switch4/1 -> Integrator2/1
  Equal1/1 -> OR/1
  Integrator2/1 -> Saturation2/1, delta_dot/1
  Switch3/1 -> Integrator3/1
  Constant12/1 -> Switch3/3
  Constant/1 -> Integrator3/2
  Constant13/1 -> Switch4/3
  Saturation1/1 -> Equal1/1, delta/1
  delta_dot_dot/1 -> Sign1/1, Saturation/1
  Constant1/1 -> Integrator2/2
  Sign1/1 -> NotEqual/2
  Sign/1 -> NotEqual/1
  NotEqual/1 -> OR/2
  OR/1 -> Switch4/2, Switch3/2
  Saturation/1 -> Switch4/1
  Saturation2/1 -> Switch3/1

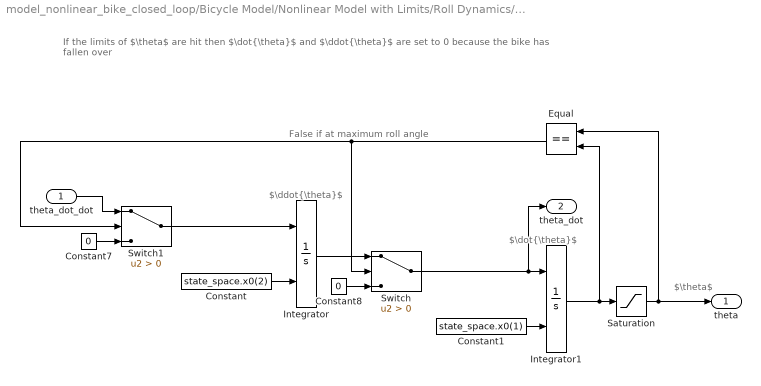
== system model_nonlinear_bike_closed_loop/Bicycle Model/Nonlinear Model with Limits/Roll Dynamics/Subsystem1 ==
  note: If the limits of $\theta$ are hit then $\dot{\theta}$ and $\ddot{\theta}$ are set to 0 because the bike has fallen over
  note: False if at maximum roll angle
  note: $\theta$
  note: $\dot{\theta}$
  note: $\ddot{\theta}$
  theta_dot_dot : Inport
  Constant : Constant  Value=state_space.x0(2)
  Constant1 : Constant  Value=state_space.x0(1)
  Constant7 : Constant  Value=0
  Constant8 : Constant  Value=0
  Equal : RelationalOperator  Operator===  OutDataTypeStr=boolean  RndMeth=Simplest
  Integrator : Integrator  InitialConditionSource=external
  Integrator1 : Integrator  InitialConditionSource=external
  Saturation : Saturate  UpperLimit=model_settings.limit_roll_angle_max  LowerLimit=model_settings.limit_roll_angle_min
  Switch : Switch  Criteria=u2 > Threshold
  Switch1 : Switch  Criteria=u2 > Threshold
  theta : Outport
  theta_dot : Outport  Port=2
  wires:
  Integrator/1 -> Switch/1
  Constant1/1 -> Integrator1/2
  Constant7/1 -> Switch1/3
  Integrator1/1 -> Saturation/1, Equal/2
  Equal/1 -> Switch/2, Switch1/2
  Constant/1 -> Integrator/2
  Constant8/1 -> Switch/3
  Saturation/1 -> Equal/1, theta/1
  theta_dot_dot/1 -> Switch1/1
  Switch/1 -> theta_dot/1, Integrator1/1
  Switch1/1 -> Integrator/1

== system model_nonlinear_bike_closed_loop/Bicycle Model/Nonlinear Model with Limits/Roll Dynamics/Subsystem2 ==
  v : Inport
  delta_dot : Inport  Port=2
  Constant1 : Constant  Value=bike.rearlength
  Constant2 : Constant  Value=bike.wheelbase
  Constant3 : Constant  Value=bike.height
  Divide1 : Product  Inputs=*/
  Multiply : Product  Inputs=3
  Multiply1 : Product
  out : Outport
  wires:
  Divide1/1 -> out/1
  Constant1/1 -> Multiply/1
  v/1 -> Multiply/2
  Constant2/1 -> Multiply1/1
  Multiply/1 -> Divide1/1
  Multiply1/1 -> Divide1/2
  Constant3/1 -> Multiply1/2
  delta_dot/1 -> Multiply/3

== system model_nonlinear_bike_closed_loop/Bicycle Model/Nonlinear Model with Limits/Roll Dynamics/Subsystem3 ==
  v : Inport
  delta : Inport  Port=2
  Constant4 : Constant  Value=bike.height
  Constant6 : Constant  Value=bike.wheelbase
  Divide2 : Product  Inputs=**/
  Multiply2 : Product
  Square : Math  Operator=square  SaturateOnIntegerOverflow=on
  out : Outport
  wires:
  delta/1 -> Divide2/2
  Constant6/1 -> Multiply2/1
  Square/1 -> Divide2/1
  Multiply2/1 -> Divide2/3
  v/1 -> Square/1
  Constant4/1 -> Multiply2/2
  Divide2/1 -> out/1

== system model_nonlinear_bike_closed_loop/Bicycle Model/Nonlinear Model with Limits/Roll Dynamics/Subsystem4 ==
  theta : Inport
  Constant : Constant  Value=bike.height
  Divide : Product  Inputs=**/
  Gravity : Constant  Value=parameters.g
  Sin : Trigonometry
  out : Outport
  wires:
  Gravity/1 -> Divide/1
  Divide/1 -> out/1
  theta/1 -> Sin/1
  Constant/1 -> Divide/3
  Sin/1 -> Divide/2

== system model_nonlinear_bike_closed_loop/Bicycle Model/Nonlinear Model with Limits/Velocity Dynamics/Subsystem ==
  note: $T$
  T : Inport
  Constant5 : Constant  Value=bike.mass
  Divide3 : Product  Inputs=*/
  Multiply3 : Product
  Rear wheel : Constant  Value=bike.diamW1
  Saturation : Saturate  UpperLimit=model_settings.limit_torque_max  LowerLimit=model_settings.limit_torque_min  ZeroCross=off
  out : Outport
  wires:
  Multiply3/1 -> Divide3/2
  Rear wheel/1 -> Multiply3/2
  Constant5/1 -> Multiply3/1
  T/1 -> Saturation/1
  Divide3/1 -> out/1
  Saturation/1 -> Divide3/1

== system model_nonlinear_bike_closed_loop/Bicycle Model/Nonlinear Model with Limits/Velocity Dynamics/Subsystem5 ==
  v : Inport
  Constant14 : Constant  Value=0
  Constant17 : Constant  Value=model_settings.simulate_friction
  Constant9 : Constant  Value=bike.velocity_friction
  Multiply4 : Product
  Switch5 : Switch  Criteria=u2 > Threshold
  out : Outport
  wires:
  Constant14/1 -> Switch5/3
  Multiply4/1 -> Switch5/1
  Constant17/1 -> Switch5/2
  Constant9/1 -> Multiply4/1
  v/1 -> Multiply4/2
  Switch5/1 -> out/1

== system model_nonlinear_bike_closed_loop/Bicycle Model/Nonlinear Model with Limits/Velocity Dynamics/Subsystem6 ==
  v : Inport
  Abs : Abs  ZeroCross=off
  Constant10 : Constant  Value=bike.constant_friction
  Constant11 : Constant  Value=0
  Constant15 : Constant  Value=0
  Constant16 : Constant  Value=model_settings.simulate_friction
  Multiply5 : Product
  Sign : Signum  ZeroCross=off
  Switch2 : Switch  Criteria=u2 > Threshold
  Switch6 : Switch  Criteria=u2 > Threshold
  out : Outport
  wires:
  Constant10/1 -> Switch2/1
  Constant11/1 -> Switch2/3
  Multiply5/1 -> Switch6/1
  Constant15/1 -> Switch6/3
  Sign/1 -> Abs/1, Multiply5/2
  Switch2/1 -> Multiply5/1
  Abs/1 -> Switch2/2
  Constant16/1 -> Switch6/2
  Switch6/1 -> out/1
  v/1 -> Sign/1

== system model_nonlinear_bike_closed_loop/Bicycle Model/Nonlinear Model with Limits/Velocity Dynamics/Subsystem7 ==
  a : Inport
  Constant : Constant  Value=state_space.x0(5)
  Integrator4 : Integrator  InitialConditionSource=external
  v : Outport
  wires:
  Constant/1 -> Integrator4/2
  Integrator4/1 -> v/1
  a/1 -> Integrator4/1

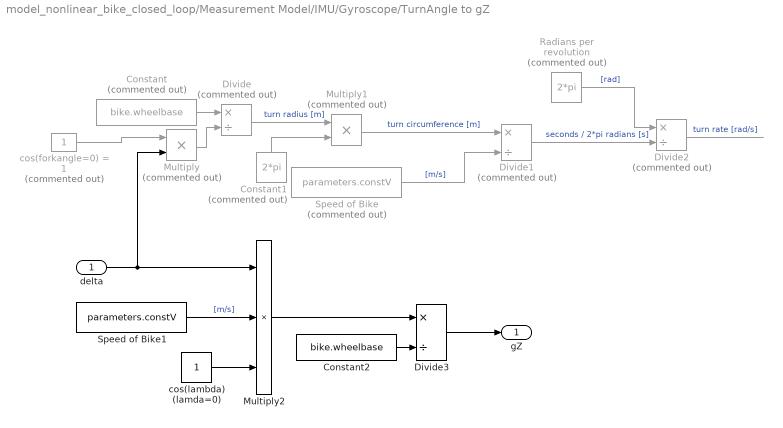
== system model_nonlinear_bike_closed_loop/Measurement Model/IMU/Gyroscope/TurnAngle to gZ ==
  delta : Inport
  Constant : Constant  Commented=on  Value=bike.wheelbase
  Constant1 : Constant  Commented=on  Value=2*pi
  Constant2 : Constant  Value=bike.wheelbase
  Divide : Product  Commented=on  Inputs=*/
  Divide1 : Product  Commented=on  Inputs=*/
  Divide2 : Product  Commented=on  Inputs=*/
  Divide3 : Product  Inputs=*/
  Multiply : Product  Commented=on
  Multiply1 : Product  Commented=on
  Multiply2 : Product  Inputs=3
  Radians per revolution : Constant  Commented=on  Value=2*pi
  Speed of Bike : Constant  Commented=on  Value=parameters.constV
  Speed of Bike1 : Constant  Value=parameters.constV
  cos(forkangle=0) = 1 : Constant  Commented=on
  cos(lambda) (lamda=0) : Constant
  gZ : Outport
  wires:
  Constant/1 -> Divide/1
  Multiply/1 -> Divide/2
  cos(forkangle=0) = 1/1 -> Multiply/1
  delta/1 -> Multiply/2, Multiply2/1
  Divide/1 -> Multiply1/1  "turn radius [m]"
  Constant1/1 -> Multiply1/2
  Multiply1/1 -> Divide1/1  "turn circumference [m]"
  Speed of Bike/1 -> Divide1/2  "[m/s]"
  Divide1/1 -> Divide2/2  "seconds / 2*pi radians [s]"
  Radians per revolution/1 -> Divide2/1  "[rad]"
  Divide2/1 -> ?  "turn rate [rad/s]"
  Speed of Bike1/1 -> Multiply2/2  "[m/s]"
  Multiply2/1 -> Divide3/1
  cos(lambda) (lamda=0)/1 -> Multiply2/3
  Constant2/1 -> Divide3/2
  Divide3/1 -> gZ/1

== matlab function model_nonlinear_bike_closed_loop/Controller/Dynamic controller/MATLAB Function ==
  data: feedback output; vmin input; vmax input; state input
function feedback = fcn(vmin,vmax,state)

v = state(5);

K = k_lookup(v,vmin,vmax);

feedback = -K*state;

== matlab function model_nonlinear_bike_closed_loop/Monitor/Convert statespace to worldframe/Convert Statespace to World frame ==
  data: orientation_n input; delta input; velocity input; Vel_FW output
function Vel_FW   = fcn(orientation_n,delta,velocity)
% This converts the two variables delta and v from the statespace 
% [delta,ddelta,theta,dtheta,v] into global position coordinates.
%delta = -delta;
% Shorten the inputnames
psi = orientation_n;
v = velocity;

% Forward kinematics from World frame to inner frame 
H_IG = [cos(psi),   sin(psi),   0;...
        -sin(psi),  cos(psi),   0;...
        0,          0,          1];    

H_FR = [cos(delta),   sin(delta),   0;...
        -sin(delta),  cos(delta),   0;...
        0,          0,          1];    
    
Vel_FI = [   v;                  ...
            v*tan(delta);       ...% The minus sign is just so that if the 
            1               ];      % angle is negative it should turn left 
                                    % Its estetics         
                               
VelFW = H_IG*H_FR\Vel_FI;                                   % are odd
Vel_FW = VelFW(1:2);

end

== matlab function model_nonlinear_bike_closed_loop/Trajectory/MATLAB Function ==
  data: t input; v output; t_case input; v0 input
function v = fcn(t,t_case, v0)


switch t_case
    case 1
        v = v0;
    case 2
        if t < 15
            v = v0;
        elseif t < 35
            v = v0 - v0/20*(t-15);
        else
            v = 0;
        end
    case 3
        if t < 5
            v = v0;
        elseif t < 15
            v = v0 + v0/20*(t-5);
        elseif t < 20
            v = v0 + v0/2;
        elseif t < 30
            v = 1.5*v0 - v0/20*(t-20);
        else
            v = v0;
        end
    case 4
        if t < 5
            v = v0;
        elseif t < 15
            v = v0 + v0/20*(t-5);
        elseif t < 20
            v = v0 + v0/2;
        elseif t < 40
            v = 1.5*v0 - v0/20*(t-20);
        elseif t < 45
            v = 0.5*v0;
        elseif t < 55
            v = 0.5*v0 - v0/20*(t-45);
        else
            v = 0;
        end
    case 5
        if t < 5
            v = v0;
        elseif t < 9
            v = v0 - v0/40*(t-5);
        else
            v = v0 - v0/40*(4);
        end
    case 6
        if t < 10
            v = v0 + v0/5*t;
        else
            v = 3*v0;
        end
    otherwise
        v = v0;
end

== matlab function model_nonlinear_bike_closed_loop/State Observer/Simulink Function - State Transition/MATLAB SFunction ==
  data: xhat input; next_xhat output
function next_xhat = StateTransferFcn(xhat)
% Input should be the entire state vector 7x1
next_xhat = EKF_TransferFcn(xhat);

== matlab function model_nonlinear_bike_closed_loop/State Observer/Simulink Function - Jacobian State Transition /MATLAB Function ==
  data: xhat input; A output
function A = StateTransferJacobian(xhat)
% The input should only be the states delta, d_delta and v
A = EKF_TransferFcnJacobian(xhat);

== matlab function model_nonlinear_bike_closed_loop/Monitor/Convert statespace to worldframe/MATLAB Function ==
  data: orientation input; Pos_frontwheel input; Pos_BW output
function Pos_BW = fcn(orientation,Pos_frontwheel)

psi = orientation;

H_IG = [cos(psi),   sin(psi),   0;...
        -sin(psi),  cos(psi),   0;...
        0,          0,          1];    

H_BF = [1, 0, 1.1;...
        0, 1, 0;...
        0, 0, 1];

PosBW = H_IG*(H_BF\(H_IG\[Pos_frontwheel;1])); 

Pos_BW = PosBW(1:2);
